simulink model "SPIPotentiometer"  (R2016b)
settings: Solver=FixedStepAuto  StartTime=0.0  StopTime=inf  FixedStep=Tsa  RelTol=1e-3  EnableMultiTasking=on
values from neighbouring files (symbols this model uses):
  Tsa = 1    [TempControlSysId.mat]
libraries: EEE481Arduino x3
settings Model: ExtModeTrigDuration=2  Creator=rsjoshi1  LastModifiedBy=rsjoshi1
settings OptimizationCC: LifeSpan=1  MaxStackSize=64
settings DebuggingCC: SFUnexpectedBacktrackingDiag=warning  SFNoUnconditionalDefaultTransitionDiag=warning  SFExecutionAtInitializationDiag=none
settings HardwareCC: ProdBitPerPointer=32  ProdBitPerSizeT=32  ProdBitPerPtrDiffT=32  ProdLargestAtomicInteger=Long  ProdLargestAtomicFloat=Double  ProdWordSize=32  ProdHWDeviceType=ARM Compatible->ARM Cortex
settings RTWCC: SystemTargetFile=ert.tlc  HardwareBoard=Arduino Due  TLCOptions=-aInlineSetEventsForThisBaseRateFcn=TLC_FALSE -aSuppressMultiTaskScheduler=TLC_FALSE -aRateBasedStepFcn=1  TemplateMakefile=ert_default_tmf  Description=Embedded Coder  GenerateReport=on  Toolchain=Arduino ARM v1.6.7  BuildConfiguration=Faster Runs  IncludeHyperlinkInReport=on  LaunchReport=on  GenerateTraceInfo=on  GenerateTraceReport=on  GenerateTraceReportSl=on  GenerateTraceReportSf=on  GenerateTraceReportEml=on
settings CodeAppCC: ForceParamTrailComments=on  IgnoreCustomStorageClasses=off  OperatorAnnotations=on  SimulinkDataObjDesc=on  SFDataObjDesc=on  MATLABFcnDesc=on  InsertBlockDesc=on  MATLABSourceComments=on
settings ERTTargetCC: SupportContinuousTime=on  SupportVariableSizeSignals=on
settings ConfigComp: CovMetricSettings=dw  CovHtmlReporting=on  CovSaveCumulativeToWorkspaceVar=on  CovSaveSingleToWorkspaceVar=on  CovExternalEMLEnable=off

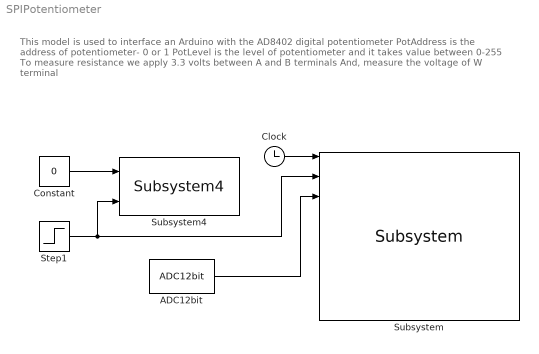
== system SPIPotentiometer ==
  note: This model is used to interface an Arduino with the AD8402 digital potentiometer
      | PotAddress is the address of potentiometer- 0 or 1
      | PotLevel is the level of potentiometer and it takes value between 0-255
      | To measure resistance we apply 3.3 volts between A and B terminals
      | And, measure the voltage of W terminal
  ADC12bit : EEE481Arduino/ADC12bit  pinNum=7  Tsa=Tsa
  Clock : Clock
  Constant : Constant  Value=0
  Step1 : Step  Time=50  Before=10  After=250  SampleTime=Tsa
  Subsystem : EEE481Arduino/Subsystem  Tsa=Tsa  rate=0  per=4
  Subsystem4 : EEE481Arduino/Subsystem4  CS=53  Tsa=Tsa
  wires:
  Clock/1 -> Subsystem/1
  ADC12bit/1 -> Subsystem/3
  Constant/1 -> Subsystem4/1
  Step1/1 -> Subsystem/2, Subsystem4/2
